simulink model "parallelreceiver"  (R2013a)
settings: Solver=ode45  StartTime=0.0  StopTime=10.0  RelTol=1e-3
libraries: commcrc2 x2, commrandsrc2 x1
settings Model: Creator=chenhr  LastModifiedBy=chenhr

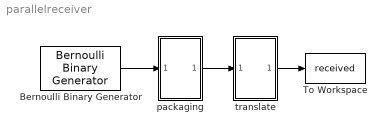
== system parallelreceiver ==
  Bernoulli Binary Generator : commrandsrc2/Bernoulli Binary Generator  P=0.5  seed=61  Ts=0.00015625  frameBased=on  sampPerFrame=64  orient=off  outDataType=double
  To Workspace : ToWorkspace  VariableName=received  SampleTime=-1  SaveFormat=Timeseries
  packaging : Subsystem
  translate : Subsystem
  wires:
  Bernoulli Binary Generator/1 -> packaging/1(In1)
  packaging/1(Out1) -> translate/1(In1)
  translate/1(Out1) -> To Workspace/1

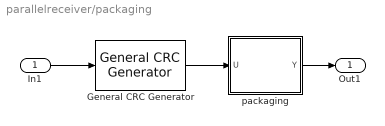
== system parallelreceiver/packaging ==
  In1 : Inport
  General CRC Generator : commcrc2/General CRC Generator  genPoly=[1 0 0 0 1 0 0 0 0 0 0 1 0 0 0 0 1]  iniStates=0  directMethod=off  reflectInputBytes=off  reflectChecksums=off  finalXOR=0  numChecksums=1
  packaging : MATLAB Function  TreatAsAtomicUnit=on  SystemSampleTime=0.01
  Out1 : Outport
  wires:
  packaging/1(Y) -> Out1/1
  In1/1 -> General CRC Generator/1
  General CRC Generator/1 -> packaging/1(U)

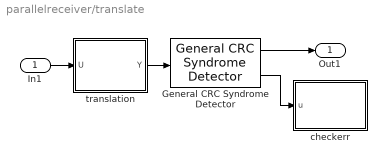
== system parallelreceiver/translate ==
  In1 : Inport
  General CRC Syndrome Detector : commcrc2/General CRC Syndrome Detector  genPoly=[1 0 0 0 1 0 0 0 0 0 0 1 0 0 0 0 1]  iniStates=0  directMethod=off  reflectInputBytes=off  reflectChecksums=off  finalXOR=0  numChecksums=1
  checkerr : MATLAB Function  TreatAsAtomicUnit=on
  translation : MATLAB Function  TreatAsAtomicUnit=on  SystemSampleTime=0.01
  Out1 : Outport
  wires:
  In1/1 -> translation/1(U)
  translation/1(Y) -> General CRC Syndrome Detector/1
  General CRC Syndrome Detector/2 -> checkerr/1(u)
  General CRC Syndrome Detector/1 -> Out1/1

== matlab function parallelreceiver/packaging/packaging ==
  data: Y output; U input
function Y   = fcn(U)
N = length(U);
Y = zeros(N * 2 + 22, 1);
Y(1:18, 1) = [1, 0, 1, 1, 0, 0, 0, 1, 1, 1, 0, 0, 0, 1, 0, 1, 0, 1]';
for i = 1:N
    if U(i) == 0
        Y(17 + i * 2) = 0;
        Y(18 + i * 2) = 1;
    else
        Y(17 + i * 2) = 1;
        Y(18 + i * 2) = 0;
    end
end
Y((19 + 2 * N):(22 + 2 * N), 1) = [0, 0, 1, 1]';
end

== matlab function parallelreceiver/translate/translation ==
  data: U input; Y output
function Y  = fcn(U)
head = [1, 0, 1, 1, 0, 0, 0, 1, 1, 1, 0, 0, 0, 1, 0, 1, 0, 1];
H = length(head);
tail = [0, 0, 1, 1];
N = length(U) - H - length(tail);
if mod(N, 2) ~= 0
    Y = zeros(N / 2, 1);
    return;
end
N = N / 2;
Y = zeros(N,1);
for t = 1:H
    if U(t) ~= head(t)
        return;
    end
end
for t = 1:N
    if (U(H + t * 2 - 1) == 0) && (U(H + t * 2) == 1)
        Y(t) = 0;
    else if (U(H + t * 2 - 1) == 1) && (U(H + t * 2) == 0)
            Y(t) = 1;
        else
            return;
        end
    end
end

== matlab function parallelreceiver/translate/checkerr ==
  data: u input
function fcn(u)
if u ~= 0
    fprintf('CRC Verification Failed!\n');
end
